simulink model "Final_V620140905h5b_fuben1"  (Simulink 7.9)
settings: Solver=FixedStepDiscrete  StartTime=0.0  StopTime=1  FixedStep=Auto  RelTol=1e-3
undefined symbols (not defined in the file or in its folder): Down, Up
libraries: tiiqmathlib x157, idelinklib_common x83, c2833xlib x37, simulink x12, c28xdmclib x12, c280xlib x7, simulink_extras x4, commutil2 x2, idelinklib_tgtpref x1, idelinklib_ticcs x1
(part 4 of 7)

== system Final_V620140905h5b_fuben1/action for state1 ==
  note: The fourth one is for load switch 0 is on
  note: The last one is for protect 0 is protect
  note: The sixth one is for Q2 on singal, 0 is on when the Q2 wants to be turned off, the i/o must be set to 1
  note: The third one is for Q2 off singal, 0 is off when the Q2 wants to be turned on, the i/o must be set to 1
  Action Port : ActionPort  ActionType=case
  Constant1 : Constant  Priority=1  Value=0  OutDataTypeStr=boolean
  Constant6 : Constant  Priority=1  Value=[1 1 1 1 1 0 1 1]  OutDataTypeStr=int8
  Digital Output : c2833xlib/Digital Output  Tag=1  Priority=2  GPIO_Number=GPIO8~GPIO15  GPIO_Bit0=off  GPIO_BIT0_Toggle=off  GPIO_Bit1=off  GPIO_BIT1_Toggle=off  GPIO_Bit2=off  GPIO_BIT2_Toggle=off  GPIO_Bit3=off  GPIO_BIT3_Toggle=off  GPIO_Bit4=on  GPIO_BIT4_Toggle=off  GPIO_Bit5=off  GPIO_BIT5_Toggle=off  GPIO_Bit6=off  GPIO_BIT6_Toggle=off  GPIO_Bit7=off  GPIO_BIT7_Toggle=off
  Out : Outport
  wires:
  Constant1/1 -> Digital Output/1
  Constant6/1 -> Out/1

== system Final_V620140905h5b_fuben1/action for state10 ==
  note: The third one is for Q2 off singal, 0 is off when the Q2 wants to be turned on, the i/o must be set to 1
  note: The sixth one is for Q2 on singal, 0 is on when the Q2 wants to be turned off, the i/o must be set to 1
  note: The last one is for protect 0 is protect
  note: The fourth one is for load switch 0 is on
  K : Inport
  Action Port : ActionPort  ActionType=case
  Constant1 : Constant  Priority=1  Value=0  OutDataTypeStr=boolean
  Constant3 : Constant  Priority=1  Value=[1 0 0 1 1 1 1 0]  OutDataTypeStr=int8
  Constant6 : Constant  Priority=1  Value=[1 1 1 1 1 1 1 0]  OutDataTypeStr=int8
  Digital Output : c2833xlib/Digital Output  Tag=1  Priority=2  GPIO_Number=GPIO8~GPIO15  GPIO_Bit0=off  GPIO_BIT0_Toggle=off  GPIO_Bit1=off  GPIO_BIT1_Toggle=off  GPIO_Bit2=off  GPIO_BIT2_Toggle=off  GPIO_Bit3=off  GPIO_BIT3_Toggle=off  GPIO_Bit4=on  GPIO_BIT4_Toggle=off  GPIO_Bit5=off  GPIO_BIT5_Toggle=off  GPIO_Bit6=off  GPIO_BIT6_Toggle=off  GPIO_Bit7=off  GPIO_BIT7_Toggle=off
  Switch1 : Switch  Criteria=u2 > Threshold  SaturateOnIntegerOverflow=on  InputSameDT=on
  Out : Outport
  wires:
  Constant1/1 -> Digital Output/1
  Switch1/1 -> Out/1
  K/1 -> Switch1/2
  Constant3/1 -> Switch1/1
  Constant6/1 -> Switch1/3

== system Final_V620140905h5b_fuben1/action for state11 ==
  note: The fourth one is for load switch 0 is on
  note: The last one is for protect 0 is protect
  note: The sixth one is for Q2 on singal, 0 is on when the Q2 wants to be turned off, the i/o must be set to 1
  note: The third one is for Q2 off singal, 0 is off when the Q2 wants to be turned on, the i/o must be set to 1
  Action Port : ActionPort  ActionType=case
  Constant1 : Constant  Priority=1  Value=0  OutDataTypeStr=boolean
  Constant6 : Constant  Priority=1  Value=[1 1 1 1 1 1 0 1]  OutDataTypeStr=int8
  Digital Output : c2833xlib/Digital Output  Tag=1  Priority=2  GPIO_Number=GPIO8~GPIO15  GPIO_Bit0=off  GPIO_BIT0_Toggle=off  GPIO_Bit1=off  GPIO_BIT1_Toggle=off  GPIO_Bit2=off  GPIO_BIT2_Toggle=off  GPIO_Bit3=off  GPIO_BIT3_Toggle=off  GPIO_Bit4=on  GPIO_BIT4_Toggle=off  GPIO_Bit5=off  GPIO_BIT5_Toggle=off  GPIO_Bit6=off  GPIO_BIT6_Toggle=off  GPIO_Bit7=off  GPIO_BIT7_Toggle=off
  Out : Outport
  wires:
  Constant1/1 -> Digital Output/1
  Constant6/1 -> Out/1

== system Final_V620140905h5b_fuben1/action for state12 ==
  note: The third one is for Q2 off singal, 0 is off when the Q2 wants to be turned on, the i/o must be set to 1
  note: The sixth one is for Q2 on singal, 0 is on when the Q2 wants to be turned off, the i/o must be set to 1
  note: The last one is for protect 0 is protect
  note: The fourth one is for load switch 0 is on
  Action Port : ActionPort  ActionType=case
  Constant1 : Constant  Priority=1  Value=0  OutDataTypeStr=boolean
  Constant6 : Constant  Priority=1  Value=[1 1 1 1 1 0 1 1]  OutDataTypeStr=int8
  Digital Output : c2833xlib/Digital Output  Tag=1  Priority=2  GPIO_Number=GPIO8~GPIO15  GPIO_Bit0=off  GPIO_BIT0_Toggle=off  GPIO_Bit1=off  GPIO_BIT1_Toggle=off  GPIO_Bit2=off  GPIO_BIT2_Toggle=off  GPIO_Bit3=off  GPIO_BIT3_Toggle=off  GPIO_Bit4=on  GPIO_BIT4_Toggle=off  GPIO_Bit5=off  GPIO_BIT5_Toggle=off  GPIO_Bit6=off  GPIO_BIT6_Toggle=off  GPIO_Bit7=off  GPIO_BIT7_Toggle=off
  Out : Outport
  wires:
  Constant1/1 -> Digital Output/1
  Constant6/1 -> Out/1

== system Final_V620140905h5b_fuben1/action for state2 ==
  note: The fourth one is for load switch 0 is on
  note: The last one is for protect 0 is protect
  note: The sixth one is for Q2 on singal, 0 is on when the Q2 wants to be turned off, the i/o must be set to 1
  note: The third one is for Q2 off singal, 0 is off when the Q2 wants to be turned on, the i/o must be set to 1
  Action Port : ActionPort  ActionType=case
  Constant1 : Constant  Priority=1  Value=0  OutDataTypeStr=boolean
  Constant6 : Constant  Priority=1  Value=[1 1 1 1 1 0 1 1]  OutDataTypeStr=int8
  Digital Output : c2833xlib/Digital Output  Tag=1  Priority=2  GPIO_Number=GPIO8~GPIO15  GPIO_Bit0=off  GPIO_BIT0_Toggle=off  GPIO_Bit1=off  GPIO_BIT1_Toggle=off  GPIO_Bit2=off  GPIO_BIT2_Toggle=off  GPIO_Bit3=off  GPIO_BIT3_Toggle=off  GPIO_Bit4=on  GPIO_BIT4_Toggle=off  GPIO_Bit5=off  GPIO_BIT5_Toggle=off  GPIO_Bit6=off  GPIO_BIT6_Toggle=off  GPIO_Bit7=off  GPIO_BIT7_Toggle=off
  Out : Outport
  wires:
  Constant1/1 -> Digital Output/1
  Constant6/1 -> Out/1

== system Final_V620140905h5b_fuben1/action for state3 ==
  note: The fourth one is for load switch 0 is on
  note: The last one is for protect 0 is protect
  note: The sixth one is for Q2 on singal, 0 is on when the Q2 wants to be turned off, the i/o must be set to 1
  note: The third one is for Q2 off singal, 0 is off when the Q2 wants to be turned on, the i/o must be set to 1
  Action Port : ActionPort  ActionType=case
  Constant1 : Constant  Priority=1  Value=0  OutDataTypeStr=boolean
  Constant6 : Constant  Priority=1  Value=[1 1 1 1 1 0 0 1]  OutDataTypeStr=int8
  Digital Output : c2833xlib/Digital Output  Tag=1  Priority=2  GPIO_Number=GPIO8~GPIO15  GPIO_Bit0=off  GPIO_BIT0_Toggle=off  GPIO_Bit1=off  GPIO_BIT1_Toggle=off  GPIO_Bit2=off  GPIO_BIT2_Toggle=off  GPIO_Bit3=off  GPIO_BIT3_Toggle=off  GPIO_Bit4=on  GPIO_BIT4_Toggle=off  GPIO_Bit5=off  GPIO_BIT5_Toggle=off  GPIO_Bit6=off  GPIO_BIT6_Toggle=off  GPIO_Bit7=off  GPIO_BIT7_Toggle=off
  Out : Outport
  wires:
  Constant1/1 -> Digital Output/1
  Constant6/1 -> Out/1

== system Final_V620140905h5b_fuben1/action for state5 ==
  note: Bit0:Fault=0
      | Bit1:G Connect to bus = 0
      | Bit2:
      | Bit3.Bit4:Lock switch = 0
      | Bit
  K : Inport
  Action Port : ActionPort  ActionType=case
  Constant1 : Constant  Priority=1  Value=0  OutDataTypeStr=boolean
  Constant3 : Constant  Priority=1  Value=[1 0 0 0 0 0 0 1]  OutDataTypeStr=int8
  Constant6 : Constant  Priority=1  Value=[1 1 1 0 0 0 0 1]  OutDataTypeStr=int8
  Digital Output : c2833xlib/Digital Output  Tag=1  Priority=2  GPIO_Number=GPIO8~GPIO15  GPIO_Bit0=off  GPIO_BIT0_Toggle=off  GPIO_Bit1=off  GPIO_BIT1_Toggle=off  GPIO_Bit2=off  GPIO_BIT2_Toggle=off  GPIO_Bit3=off  GPIO_BIT3_Toggle=off  GPIO_Bit4=on  GPIO_BIT4_Toggle=off  GPIO_Bit5=off  GPIO_BIT5_Toggle=off  GPIO_Bit6=off  GPIO_BIT6_Toggle=off  GPIO_Bit7=off  GPIO_BIT7_Toggle=off
  Switch1 : Switch  Criteria=u2 > Threshold  SaturateOnIntegerOverflow=on  InputSameDT=on
  Out : Outport
  wires:
  Constant1/1 -> Digital Output/1
  Switch1/1 -> Out/1
  K/1 -> Switch1/2
  Constant3/1 -> Switch1/1
  Constant6/1 -> Switch1/3

== system Final_V620140905h5b_fuben1/action for state6 ==
  note: The fourth one is for load switch 0 is on
  note: The last one is for protect 0 is protect
  note: The sixth one is for Q2 on singal, 0 is on when the Q2 wants to be turned off, the i/o must be set to 1
  note: The third one is for Q2 off singal, 0 is off when the Q2 wants to be turned on, the i/o must be set to 1
  Action Port : ActionPort  ActionType=case
  Constant1 : Constant  Priority=1  Value=0  OutDataTypeStr=boolean
  Constant6 : Constant  Priority=1  Value=[1 1 1 0 0 1 0 1]  OutDataTypeStr=int8
  Digital Output : c2833xlib/Digital Output  Tag=1  Priority=2  GPIO_Number=GPIO8~GPIO15  GPIO_Bit0=off  GPIO_BIT0_Toggle=off  GPIO_Bit1=off  GPIO_BIT1_Toggle=off  GPIO_Bit2=off  GPIO_BIT2_Toggle=off  GPIO_Bit3=off  GPIO_BIT3_Toggle=off  GPIO_Bit4=on  GPIO_BIT4_Toggle=off  GPIO_Bit5=off  GPIO_BIT5_Toggle=off  GPIO_Bit6=off  GPIO_BIT6_Toggle=off  GPIO_Bit7=off  GPIO_BIT7_Toggle=off
  Out : Outport
  wires:
  Constant1/1 -> Digital Output/1
  Constant6/1 -> Out/1

== system Final_V620140905h5b_fuben1/action for state7 ==
  note: The fourth one is for load switch 0 is on
  note: The last one is for protect 0 is protect
  note: The sixth one is for Q2 on singal, 0 is on when the Q2 wants to be turned off, the i/o must be set to 1
  note: The third one is for Q2 off singal, 0 is off when the Q2 wants to be turned on, the i/o must be set to 1
  Action Port : ActionPort  ActionType=case
  Constant1 : Constant  Priority=1  Value=0  OutDataTypeStr=boolean
  Constant6 : Constant  Priority=1  Value=[1 1 1 0 0 1 0 1]  OutDataTypeStr=int8
  Digital Output : c2833xlib/Digital Output  Tag=1  Priority=2  GPIO_Number=GPIO8~GPIO15  GPIO_Bit0=off  GPIO_BIT0_Toggle=off  GPIO_Bit1=off  GPIO_BIT1_Toggle=off  GPIO_Bit2=off  GPIO_BIT2_Toggle=off  GPIO_Bit3=off  GPIO_BIT3_Toggle=off  GPIO_Bit4=on  GPIO_BIT4_Toggle=off  GPIO_Bit5=off  GPIO_BIT5_Toggle=off  GPIO_Bit6=off  GPIO_BIT6_Toggle=off  GPIO_Bit7=off  GPIO_BIT7_Toggle=off
  Out : Outport
  wires:
  Constant1/1 -> Digital Output/1
  Constant6/1 -> Out/1

== system Final_V620140905h5b_fuben1/action for state8 ==
  note: The third one is for Q2 off singal, 0 is off when the Q2 wants to be turned on, the i/o must be set to 1
  note: The sixth one is for Q2 on singal, 0 is on when the Q2 wants to be turned off, the i/o must be set to 1
  note: The last one is for protect 0 is protect
  note: The fourth one is for load switch 0 is on
  Action Port : ActionPort  ActionType=case
  Constant1 : Constant  Priority=1  Value=0  OutDataTypeStr=boolean
  Constant5 : Constant  Priority=1  Value=[1 1 1 1 1 0 0 1]  OutDataTypeStr=int8
  Digital Output : c2833xlib/Digital Output  Tag=1  Priority=2  GPIO_Number=GPIO8~GPIO15  GPIO_Bit0=off  GPIO_BIT0_Toggle=off  GPIO_Bit1=off  GPIO_BIT1_Toggle=off  GPIO_Bit2=off  GPIO_BIT2_Toggle=off  GPIO_Bit3=off  GPIO_BIT3_Toggle=off  GPIO_Bit4=on  GPIO_BIT4_Toggle=off  GPIO_Bit5=off  GPIO_BIT5_Toggle=off  GPIO_Bit6=off  GPIO_BIT6_Toggle=off  GPIO_Bit7=off  GPIO_BIT7_Toggle=off
  Out : Outport
  wires:
  Constant1/1 -> Digital Output/1
  Constant5/1 -> Out/1

== system Final_V620140905h5b_fuben1/action for state9 ==
  note: The fourth one is for load switch 0 is on
  note: The last one is for protect 0 is protect
  note: The sixth one is for Q2 on singal, 0 is on when the Q2 wants to be turned off, the i/o must be set to 1
  note: The third one is for Q2 off singal, 0 is off when the Q2 wants to be turned on, the i/o must be set to 1
  Action Port : ActionPort  ActionType=case
  Constant1 : Constant  Priority=1  Value=0  OutDataTypeStr=boolean
  Constant6 : Constant  Priority=1  Value=[1 1 1 1 1 0 1 1]  OutDataTypeStr=int8
  Digital Output : c2833xlib/Digital Output  Tag=1  Priority=2  GPIO_Number=GPIO8~GPIO15  GPIO_Bit0=off  GPIO_BIT0_Toggle=off  GPIO_Bit1=off  GPIO_BIT1_Toggle=off  GPIO_Bit2=off  GPIO_BIT2_Toggle=off  GPIO_Bit3=off  GPIO_BIT3_Toggle=off  GPIO_Bit4=on  GPIO_BIT4_Toggle=off  GPIO_Bit5=off  GPIO_BIT5_Toggle=off  GPIO_Bit6=off  GPIO_BIT6_Toggle=off  GPIO_Bit7=off  GPIO_BIT7_Toggle=off
  Out : Outport
  wires:
  Constant1/1 -> Digital Output/1
  Constant6/1 -> Out/1

== system Final_V620140905h5b_fuben1/actrion for state4 ==
  note: The fourth one is for load switch 0 is on
  note: The last one is for protect 0 is protect
  note: The sixth one is for Q2 on singal, 0 is on when the Q2 wants to be turned off, the i/o must be set to 1
  note: The third one is for Q2 off singal, 0 is off when the Q2 wants to be turned on, the i/o must be set to 1
  K : Inport
  Action Port : ActionPort  ActionType=case
  Constant1 : Constant  Priority=1  Value=0  OutDataTypeStr=boolean
  Constant2 : Constant  Priority=1  Value=[1 0 0 0 0 1 0 1]  OutDataTypeStr=int8
  Constant6 : Constant  Priority=1  Value=[1 1 1 0 0 1 0 1]  OutDataTypeStr=int8
  Digital Output : c2833xlib/Digital Output  Tag=1  Priority=2  GPIO_Number=GPIO8~GPIO15  GPIO_Bit0=off  GPIO_BIT0_Toggle=off  GPIO_Bit1=off  GPIO_BIT1_Toggle=off  GPIO_Bit2=off  GPIO_BIT2_Toggle=off  GPIO_Bit3=off  GPIO_BIT3_Toggle=off  GPIO_Bit4=on  GPIO_BIT4_Toggle=off  GPIO_Bit5=off  GPIO_BIT5_Toggle=off  GPIO_Bit6=off  GPIO_BIT6_Toggle=off  GPIO_Bit7=off  GPIO_BIT7_Toggle=off
  Switch1 : Switch  Criteria=u2 > Threshold  SaturateOnIntegerOverflow=on  InputSameDT=on
  Out : Outport
  wires:
  Constant1/1 -> Digital Output/1
  K/1 -> Switch1/2
  Constant6/1 -> Switch1/3
  Switch1/1 -> Out/1
  Constant2/1 -> Switch1/1

== system Final_V620140905h5b_fuben1/Function-Call Subsystem1/0 ==
  Action Port : ActionPort  ActionType=case
  Constant{1,3..4,7..8} (5 alike) : Constant  Priority=1  Value=0  OutDataTypeStr=boolean
  Constant2 : Constant  Priority=1  OutDataTypeStr=boolean
  Constant5 : Constant  Priority=1  OutDataTypeStr=boolean
  Constant6 : Constant  Priority=1  OutDataTypeStr=boolean
  Mux : Mux  Inputs=8
  Out1 : Outport
  wires:
  Constant2/1 -> Mux/1
  Constant1/1 -> Mux/2
  Constant3/1 -> Mux/3
  Constant4/1 -> Mux/4
  Constant5/1 -> Mux/5
  Constant6/1 -> Mux/6
  Constant7/1 -> Mux/7
  Constant8/1 -> Mux/8
  Mux/1 -> Out1/1

== system Final_V620140905h5b_fuben1/Function-Call Subsystem1/1 ==
  Action Port : ActionPort  ActionType=case
  Constant1 : Constant  Priority=1  OutDataTypeStr=boolean
  Constant{2..3,5..8} (6 alike) : Constant  Priority=1  Value=0  OutDataTypeStr=boolean
  Constant4 : Constant  Priority=1  OutDataTypeStr=boolean
  Mux : Mux  Inputs=8
  Out1 : Outport
  wires:
  Mux/1 -> Out1/1
  Constant8/1 -> Mux/8
  Constant7/1 -> Mux/7
  Constant6/1 -> Mux/6
  Constant5/1 -> Mux/5
  Constant4/1 -> Mux/4
  Constant3/1 -> Mux/3
  Constant1/1 -> Mux/2
  Constant2/1 -> Mux/1

== system Final_V620140905h5b_fuben1/Function-Call Subsystem1/10 ==
  Action Port : ActionPort  ActionType=case
  Constant{1,3..8} (7 alike) : Constant  Priority=1  Value=0  OutDataTypeStr=boolean
  Constant2 : Constant  Priority=1  OutDataTypeStr=boolean
  Mux : Mux  Inputs=8
  Out1 : Outport
  wires:
  Mux/1 -> Out1/1
  Constant8/1 -> Mux/8
  Constant7/1 -> Mux/7
  Constant6/1 -> Mux/6
  Constant5/1 -> Mux/5
  Constant4/1 -> Mux/4
  Constant3/1 -> Mux/3
  Constant1/1 -> Mux/2
  Constant2/1 -> Mux/1

== system Final_V620140905h5b_fuben1/Function-Call Subsystem1/11 ==
  Action Port : ActionPort  ActionType=case
  Constant{1,3..4,7} (4 alike) : Constant  Priority=1  OutDataTypeStr=boolean
  Constant{2,5..6,8} (4 alike) : Constant  Priority=1  Value=0  OutDataTypeStr=boolean
  Mux : Mux  Inputs=8
  Out1 : Outport
  wires:
  Constant2/1 -> Mux/1
  Constant1/1 -> Mux/2
  Constant3/1 -> Mux/3
  Constant4/1 -> Mux/4
  Constant5/1 -> Mux/5
  Constant6/1 -> Mux/6
  Constant7/1 -> Mux/7
  Constant8/1 -> Mux/8
  Mux/1 -> Out1/1

== system Final_V620140905h5b_fuben1/Function-Call Subsystem1/12 ==
  Action Port : ActionPort  ActionType=case
  Constant{1..2,5..8} (6 alike) : Constant  Priority=1  Value=0  OutDataTypeStr=boolean
  Constant3 : Constant  Priority=1  OutDataTypeStr=boolean
  Constant4 : Constant  Priority=1  OutDataTypeStr=boolean
  Mux : Mux  Inputs=8
  Out1 : Outport
  wires:
  Mux/1 -> Out1/1
  Constant8/1 -> Mux/8
  Constant7/1 -> Mux/7
  Constant6/1 -> Mux/6
  Constant5/1 -> Mux/5
  Constant4/1 -> Mux/4
  Constant3/1 -> Mux/3
  Constant1/1 -> Mux/2
  Constant2/1 -> Mux/1

== system Final_V620140905h5b_fuben1/Function-Call Subsystem1/2 ==
  Action Port : ActionPort  ActionType=case
  Constant{1,3..4,7} (4 alike) : Constant  Priority=1  OutDataTypeStr=boolean
  Constant{2,5..6,8} (4 alike) : Constant  Priority=1  Value=0  OutDataTypeStr=boolean
  Mux : Mux  Inputs=8
  Out1 : Outport
  wires:
  Constant2/1 -> Mux/1
  Constant1/1 -> Mux/2
  Constant3/1 -> Mux/3
  Constant4/1 -> Mux/4
  Constant5/1 -> Mux/5
  Constant6/1 -> Mux/6
  Constant7/1 -> Mux/7
  Constant8/1 -> Mux/8
  Mux/1 -> Out1/1

== system Final_V620140905h5b_fuben1/Function-Call Subsystem1/3 ==
  Action Port : ActionPort  ActionType=case
  Constant{1,3..4,7} (4 alike) : Constant  Priority=1  OutDataTypeStr=boolean
  Constant{2,5..6,8} (4 alike) : Constant  Priority=1  Value=0  OutDataTypeStr=boolean
  Mux : Mux  Inputs=8
  Out1 : Outport
  wires:
  Mux/1 -> Out1/1
  Constant8/1 -> Mux/8
  Constant7/1 -> Mux/7
  Constant6/1 -> Mux/6
  Constant5/1 -> Mux/5
  Constant4/1 -> Mux/4
  Constant3/1 -> Mux/3
  Constant1/1 -> Mux/2
  Constant2/1 -> Mux/1

== system Final_V620140905h5b_fuben1/Function-Call Subsystem1/4 ==
  Action Port : ActionPort  ActionType=case
  Constant{1..3,5..8} (7 alike) : Constant  Priority=1  Value=0  OutDataTypeStr=boolean
  Constant4 : Constant  Priority=1  OutDataTypeStr=boolean
  Mux : Mux  Inputs=8
  Out1 : Outport
  wires:
  Constant2/1 -> Mux/1
  Constant1/1 -> Mux/2
  Constant3/1 -> Mux/3
  Constant4/1 -> Mux/4
  Constant5/1 -> Mux/5
  Constant6/1 -> Mux/6
  Constant7/1 -> Mux/7
  Constant8/1 -> Mux/8
  Mux/1 -> Out1/1

== system Final_V620140905h5b_fuben1/Function-Call Subsystem1/5 ==
  Action Port : ActionPort  ActionType=case
  Constant{1..3,5..6,8} (6 alike) : Constant  Priority=1  Value=0  OutDataTypeStr=boolean
  Constant4 : Constant  Priority=1  OutDataTypeStr=boolean
  Constant7 : Constant  Priority=1  OutDataTypeStr=boolean
  Mux : Mux  Inputs=8
  Out1 : Outport
  wires:
  Mux/1 -> Out1/1
  Constant8/1 -> Mux/8
  Constant7/1 -> Mux/7
  Constant6/1 -> Mux/6
  Constant5/1 -> Mux/5
  Constant4/1 -> Mux/4
  Constant3/1 -> Mux/3
  Constant1/1 -> Mux/2
  Constant2/1 -> Mux/1

== system Final_V620140905h5b_fuben1/Function-Call Subsystem1/6 ==
  Action Port : ActionPort  ActionType=case
  Constant1 : Constant  Priority=1  OutDataTypeStr=boolean
  Constant{2,5..8} (5 alike) : Constant  Priority=1  Value=0  OutDataTypeStr=boolean
  Constant3 : Constant  Priority=1  OutDataTypeStr=boolean
  Constant4 : Constant  Priority=1  OutDataTypeStr=boolean
  Mux : Mux  Inputs=8
  Out1 : Outport
  wires:
  Mux/1 -> Out1/1
  Constant8/1 -> Mux/8
  Constant7/1 -> Mux/7
  Constant6/1 -> Mux/6
  Constant5/1 -> Mux/5
  Constant4/1 -> Mux/4
  Constant3/1 -> Mux/3
  Constant1/1 -> Mux/2
  Constant2/1 -> Mux/1

== system Final_V620140905h5b_fuben1/Function-Call Subsystem1/7 ==
  Action Port : ActionPort  ActionType=case
  Constant{1,3..4,7} (4 alike) : Constant  Priority=1  OutDataTypeStr=boolean
  Constant{2,5..6,8} (4 alike) : Constant  Priority=1  Value=0  OutDataTypeStr=boolean
  Mux : Mux  Inputs=8
  Out1 : Outport
  wires:
  Constant2/1 -> Mux/1
  Constant1/1 -> Mux/2
  Constant3/1 -> Mux/3
  Constant4/1 -> Mux/4
  Constant5/1 -> Mux/5
  Constant6/1 -> Mux/6
  Constant7/1 -> Mux/7
  Constant8/1 -> Mux/8
  Mux/1 -> Out1/1

== system Final_V620140905h5b_fuben1/Function-Call Subsystem1/8 ==
  Action Port : ActionPort  ActionType=case
  Constant{1,3..4,7} (4 alike) : Constant  Priority=1  OutDataTypeStr=boolean
  Constant{2,5..6,8} (4 alike) : Constant  Priority=1  Value=0  OutDataTypeStr=boolean
  Mux : Mux  Inputs=8
  Out1 : Outport
  wires:
  Mux/1 -> Out1/1
  Constant8/1 -> Mux/8
  Constant7/1 -> Mux/7
  Constant6/1 -> Mux/6
  Constant5/1 -> Mux/5
  Constant4/1 -> Mux/4
  Constant3/1 -> Mux/3
  Constant1/1 -> Mux/2
  Constant2/1 -> Mux/1

== system Final_V620140905h5b_fuben1/Function-Call Subsystem1/9 ==
  Action Port : ActionPort  ActionType=case
  Constant{1..3,5..6,8} (6 alike) : Constant  Priority=1  Value=0  OutDataTypeStr=boolean
  Constant4 : Constant  Priority=1  OutDataTypeStr=boolean
  Constant7 : Constant  Priority=1  OutDataTypeStr=boolean
  Mux : Mux  Inputs=8
  Out1 : Outport
  wires:
  Constant2/1 -> Mux/1
  Constant1/1 -> Mux/2
  Constant3/1 -> Mux/3
  Constant4/1 -> Mux/4
  Constant5/1 -> Mux/5
  Constant6/1 -> Mux/6
  Constant7/1 -> Mux/7
  Constant8/1 -> Mux/8
  Mux/1 -> Out1/1

== system Final_V620140905h5b_fuben1/Function-Call Subsystem1/AD ==
  Read AD : Subsystem  Priority=2
  Start Conversion : Subsystem  Priority=1
  Stop Conversion : Subsystem  Priority=3

== system Final_V620140905h5b_fuben1/Function-Call Subsystem1/Current protect ==
  igdin : Inport
  Reset : Inport  Port=2
  Constant25 : Constant  Value=0  OutDataTypeStr=boolean
  Constant26 : Constant  OutDataTypeStr=boolean
  S-R Flip-Flop1 : simulink_extras/Flip Flops/S-R Flip-Flop  initial_condition=0
  Switch9 : Switch  Criteria=u2 > Threshold  Threshold=380  SaturateOnIntegerOverflow=on  InputSameDT=on
  Terminator : Terminator
  Software_I : Outport
  wires:
  Constant26/1 -> Switch9/1
  Constant25/1 -> Switch9/3
  S-R Flip-Flop1/1 -> Software_I/1
  Reset/1 -> S-R Flip-Flop1/2
  S-R Flip-Flop1/2 -> Terminator/1
  Switch9/1 -> S-R Flip-Flop1/1
  igdin/1 -> Switch9/2

== system Final_V620140905h5b_fuben1/Function-Call Subsystem1/Current protect1 ==
  igdin : Inport
  Reset : Inport  Port=2
  Constant25 : Constant  Value=0  OutDataTypeStr=boolean
  Constant26 : Constant  OutDataTypeStr=boolean
  S-R Flip-Flop1 : simulink_extras/Flip Flops/S-R Flip-Flop  initial_condition=0
  Switch9 : Switch  Criteria=u2 > Threshold  Threshold=350  SaturateOnIntegerOverflow=on  InputSameDT=on
  Terminator : Terminator
  Software_I : Outport
  wires:
  igdin/1 -> Switch9/2
  Switch9/1 -> S-R Flip-Flop1/1
  S-R Flip-Flop1/2 -> Terminator/1
  Reset/1 -> S-R Flip-Flop1/2
  S-R Flip-Flop1/1 -> Software_I/1
  Constant25/1 -> Switch9/3
  Constant26/1 -> Switch9/1

== system Final_V620140905h5b_fuben1/Function-Call Subsystem1/ION multiply1 ==
  x : Inport
  Constant2 : Constant  Value=x  OutDataTypeStr=fixdt(1,32,16)
  IQN x IQN : tiiqmathlib/IQN x IQN  multiplyOption=Multiply
  Kx : Outport
  wires:
  IQN x IQN/1 -> Kx/1
  x/1 -> IQN x IQN/1
  Constant2/1 -> IQN x IQN/2

== system Final_V620140905h5b_fuben1/Function-Call Subsystem1/ION multiply10 ==
  x : Inport
  Constant2 : Constant  Value=x  OutDataTypeStr=fixdt(1,32,16)
  IQN x IQN : tiiqmathlib/IQN x IQN  multiplyOption=Multiply
  Kx : Outport
  wires:
  IQN x IQN/1 -> Kx/1
  x/1 -> IQN x IQN/1
  Constant2/1 -> IQN x IQN/2

== system Final_V620140905h5b_fuben1/Function-Call Subsystem1/ION multiply11 ==
  x : Inport
  Constant2 : Constant  Value=x  OutDataTypeStr=fixdt(1,32,16)
  IQN x IQN : tiiqmathlib/IQN x IQN  multiplyOption=Multiply
  Kx : Outport
  wires:
  Constant2/1 -> IQN x IQN/2
  x/1 -> IQN x IQN/1
  IQN x IQN/1 -> Kx/1

== system Final_V620140905h5b_fuben1/Function-Call Subsystem1/ION multiply12 ==
  x : Inport
  Constant2 : Constant  Value=x  OutDataTypeStr=fixdt(1,32,16)
  IQN x IQN : tiiqmathlib/IQN x IQN  multiplyOption=Multiply
  Kx : Outport
  wires:
  Constant2/1 -> IQN x IQN/2
  x/1 -> IQN x IQN/1
  IQN x IQN/1 -> Kx/1

== system Final_V620140905h5b_fuben1/Function-Call Subsystem1/ION multiply13 ==
  x : Inport
  Constant2 : Constant  Value=x  OutDataTypeStr=fixdt(1,32,16)
  IQN x IQN : tiiqmathlib/IQN x IQN  multiplyOption=Multiply
  Kx : Outport
  wires:
  Constant2/1 -> IQN x IQN/2
  x/1 -> IQN x IQN/1
  IQN x IQN/1 -> Kx/1

== system Final_V620140905h5b_fuben1/Function-Call Subsystem1/ION multiply14 ==
  x : Inport
  Constant2 : Constant  Value=x  OutDataTypeStr=fixdt(1,32,16)
  IQN x IQN : tiiqmathlib/IQN x IQN  multiplyOption=Multiply
  Kx : Outport
  wires:
  IQN x IQN/1 -> Kx/1
  x/1 -> IQN x IQN/1
  Constant2/1 -> IQN x IQN/2

== system Final_V620140905h5b_fuben1/Function-Call Subsystem1/ION multiply15 ==
  x : Inport
  Constant2 : Constant  Value=x  OutDataTypeStr=fixdt(1,32,16)
  IQN x IQN : tiiqmathlib/IQN x IQN  multiplyOption=Multiply
  Kx : Outport
  wires:
  IQN x IQN/1 -> Kx/1
  x/1 -> IQN x IQN/1
  Constant2/1 -> IQN x IQN/2

== system Final_V620140905h5b_fuben1/Function-Call Subsystem1/ION multiply16 ==
  x : Inport
  Constant2 : Constant  Value=x  OutDataTypeStr=fixdt(1,32,16)
  IQN x IQN : tiiqmathlib/IQN x IQN  multiplyOption=Multiply
  Kx : Outport
  wires:
  IQN x IQN/1 -> Kx/1
  x/1 -> IQN x IQN/1
  Constant2/1 -> IQN x IQN/2

== system Final_V620140905h5b_fuben1/Function-Call Subsystem1/ION multiply17 ==
  x : Inport
  Constant2 : Constant  Value=x  OutDataTypeStr=fixdt(1,32,16)
  IQN x IQN : tiiqmathlib/IQN x IQN  multiplyOption=Multiply
  Kx : Outport
  wires:
  IQN x IQN/1 -> Kx/1
  x/1 -> IQN x IQN/1
  Constant2/1 -> IQN x IQN/2

== system Final_V620140905h5b_fuben1/Function-Call Subsystem1/ION multiply19 ==
  x : Inport
  Constant2 : Constant  Value=x  OutDataTypeStr=fixdt(1,32,16)
  IQN x IQN : tiiqmathlib/IQN x IQN  multiplyOption=Multiply
  Kx : Outport
  wires:
  IQN x IQN/1 -> Kx/1
  x/1 -> IQN x IQN/1
  Constant2/1 -> IQN x IQN/2

== system Final_V620140905h5b_fuben1/Function-Call Subsystem1/ION multiply2 ==
  x : Inport
  Constant2 : Constant  Value=x  OutDataTypeStr=fixdt(1,32,16)
  IQN x IQN : tiiqmathlib/IQN x IQN  multiplyOption=Multiply
  Kx : Outport
  wires:
  IQN x IQN/1 -> Kx/1
  x/1 -> IQN x IQN/1
  Constant2/1 -> IQN x IQN/2

== system Final_V620140905h5b_fuben1/Function-Call Subsystem1/ION multiply20 ==
  x : Inport
  Constant2 : Constant  Value=x  OutDataTypeStr=fixdt(1,32,16)
  IQN x IQN : tiiqmathlib/IQN x IQN  multiplyOption=Multiply
  Kx : Outport
  wires:
  Constant2/1 -> IQN x IQN/2
  x/1 -> IQN x IQN/1
  IQN x IQN/1 -> Kx/1

== system Final_V620140905h5b_fuben1/Function-Call Subsystem1/ION multiply21 ==
  x : Inport
  Constant2 : Constant  Value=x  OutDataTypeStr=fixdt(1,32,16)
  IQN x IQN : tiiqmathlib/IQN x IQN  multiplyOption=Multiply
  Kx : Outport
  wires:
  IQN x IQN/1 -> Kx/1
  x/1 -> IQN x IQN/1
  Constant2/1 -> IQN x IQN/2

== system Final_V620140905h5b_fuben1/Function-Call Subsystem1/ION multiply22 ==
  x : Inport
  Constant2 : Constant  Value=x  OutDataTypeStr=fixdt(1,32,16)
  IQN x IQN : tiiqmathlib/IQN x IQN  multiplyOption=Multiply
  Kx : Outport
  wires:
  IQN x IQN/1 -> Kx/1
  x/1 -> IQN x IQN/1
  Constant2/1 -> IQN x IQN/2

== system Final_V620140905h5b_fuben1/Function-Call Subsystem1/ION multiply23 ==
  x : Inport
  Constant2 : Constant  Value=x  OutDataTypeStr=fixdt(1,32,16)
  IQN x IQN : tiiqmathlib/IQN x IQN  multiplyOption=Multiply
  Kx : Outport
  wires:
  Constant2/1 -> IQN x IQN/2
  x/1 -> IQN x IQN/1
  IQN x IQN/1 -> Kx/1

== system Final_V620140905h5b_fuben1/Function-Call Subsystem1/ION multiply24 ==
  x : Inport
  Constant2 : Constant  Value=x  OutDataTypeStr=fixdt(1,32,16)
  IQN x IQN : tiiqmathlib/IQN x IQN  multiplyOption=Multiply
  Kx : Outport
  wires:
  IQN x IQN/1 -> Kx/1
  x/1 -> IQN x IQN/1
  Constant2/1 -> IQN x IQN/2

== system Final_V620140905h5b_fuben1/Function-Call Subsystem1/ION multiply25 ==
  x : Inport
  Constant2 : Constant  Value=x  OutDataTypeStr=fixdt(1,32,16)
  IQN x IQN : tiiqmathlib/IQN x IQN  multiplyOption=Multiply
  Kx : Outport
  wires:
  Constant2/1 -> IQN x IQN/2
  x/1 -> IQN x IQN/1
  IQN x IQN/1 -> Kx/1

== system Final_V620140905h5b_fuben1/Function-Call Subsystem1/ION multiply26 ==
  x : Inport
  Constant2 : Constant  Value=x  OutDataTypeStr=fixdt(1,32,16)
  IQN x IQN : tiiqmathlib/IQN x IQN  multiplyOption=Multiply
  Kx : Outport
  wires:
  IQN x IQN/1 -> Kx/1
  x/1 -> IQN x IQN/1
  Constant2/1 -> IQN x IQN/2

== system Final_V620140905h5b_fuben1/Function-Call Subsystem1/ION multiply27 ==
  x : Inport
  Constant2 : Constant  Value=x  OutDataTypeStr=fixdt(1,32,16)
  IQN x IQN : tiiqmathlib/IQN x IQN  multiplyOption=Multiply
  Kx : Outport
  wires:
  IQN x IQN/1 -> Kx/1
  x/1 -> IQN x IQN/1
  Constant2/1 -> IQN x IQN/2

== system Final_V620140905h5b_fuben1/Function-Call Subsystem1/ION multiply28 ==
  x : Inport
  Constant2 : Constant  Value=x  OutDataTypeStr=fixdt(1,32,16)
  IQN x IQN : tiiqmathlib/IQN x IQN  multiplyOption=Multiply
  Kx : Outport
  wires:
  Constant2/1 -> IQN x IQN/2
  x/1 -> IQN x IQN/1
  IQN x IQN/1 -> Kx/1

== system Final_V620140905h5b_fuben1/Function-Call Subsystem1/ION multiply29 ==
  x : Inport
  Constant2 : Constant  Value=x  OutDataTypeStr=fixdt(1,32,16)
  IQN x IQN : tiiqmathlib/IQN x IQN  multiplyOption=Multiply
  Kx : Outport
  wires:
  Constant2/1 -> IQN x IQN/2
  x/1 -> IQN x IQN/1
  IQN x IQN/1 -> Kx/1

== system Final_V620140905h5b_fuben1/Function-Call Subsystem1/ION multiply3 ==
  x : Inport
  Constant2 : Constant  Value=x  OutDataTypeStr=fixdt(1,32,16)
  IQN x IQN : tiiqmathlib/IQN x IQN  multiplyOption=Multiply
  Kx : Outport
  wires:
  Constant2/1 -> IQN x IQN/2
  x/1 -> IQN x IQN/1
  IQN x IQN/1 -> Kx/1

== system Final_V620140905h5b_fuben1/Function-Call Subsystem1/ION multiply30 ==
  x : Inport
  Constant2 : Constant  Value=x  OutDataTypeStr=fixdt(1,32,16)
  IQN x IQN : tiiqmathlib/IQN x IQN  multiplyOption=Multiply
  Kx : Outport
  wires:
  IQN x IQN/1 -> Kx/1
  x/1 -> IQN x IQN/1
  Constant2/1 -> IQN x IQN/2

== system Final_V620140905h5b_fuben1/Function-Call Subsystem1/ION multiply31 ==
  x : Inport
  Constant2 : Constant  Value=x  OutDataTypeStr=fixdt(1,32,16)
  IQN x IQN : tiiqmathlib/IQN x IQN  multiplyOption=Multiply
  Kx : Outport
  wires:
  IQN x IQN/1 -> Kx/1
  x/1 -> IQN x IQN/1
  Constant2/1 -> IQN x IQN/2

== system Final_V620140905h5b_fuben1/Function-Call Subsystem1/ION multiply32 ==
  x : Inport
  Constant2 : Constant  Value=x  OutDataTypeStr=fixdt(1,32,16)
  IQN x IQN : tiiqmathlib/IQN x IQN  multiplyOption=Multiply
  Kx : Outport
  wires:
  Constant2/1 -> IQN x IQN/2
  x/1 -> IQN x IQN/1
  IQN x IQN/1 -> Kx/1

== system Final_V620140905h5b_fuben1/Function-Call Subsystem1/ION multiply33 ==
  x : Inport
  Constant2 : Constant  Value=x  OutDataTypeStr=fixdt(1,32,16)
  IQN x IQN : tiiqmathlib/IQN x IQN  multiplyOption=Multiply
  Kx : Outport
  wires:
  Constant2/1 -> IQN x IQN/2
  x/1 -> IQN x IQN/1
  IQN x IQN/1 -> Kx/1

== system Final_V620140905h5b_fuben1/Function-Call Subsystem1/ION multiply34 ==
  x : Inport
  Constant2 : Constant  Value=x  OutDataTypeStr=fixdt(1,32,16)
  IQN x IQN : tiiqmathlib/IQN x IQN  multiplyOption=Multiply
  Kx : Outport
  wires:
  Constant2/1 -> IQN x IQN/2
  x/1 -> IQN x IQN/1
  IQN x IQN/1 -> Kx/1

== system Final_V620140905h5b_fuben1/Function-Call Subsystem1/ION multiply35 ==
  x : Inport
  Constant2 : Constant  Value=x  OutDataTypeStr=fixdt(1,32,16)
  IQN x IQN : tiiqmathlib/IQN x IQN  multiplyOption=Multiply
  Kx : Outport
  wires:
  IQN x IQN/1 -> Kx/1
  x/1 -> IQN x IQN/1
  Constant2/1 -> IQN x IQN/2

== system Final_V620140905h5b_fuben1/Function-Call Subsystem1/ION multiply36 ==
  x : Inport
  Constant2 : Constant  Value=x  OutDataTypeStr=fixdt(1,32,16)
  IQN x IQN : tiiqmathlib/IQN x IQN  multiplyOption=Multiply
  Kx : Outport
  wires:
  IQN x IQN/1 -> Kx/1
  x/1 -> IQN x IQN/1
  Constant2/1 -> IQN x IQN/2

== system Final_V620140905h5b_fuben1/Function-Call Subsystem1/ION multiply39 ==
  x : Inport
  Constant2 : Constant  Value=x  OutDataTypeStr=Inherit: Inherit via back propagation
  IQN x IQN : tiiqmathlib/IQN x IQN  multiplyOption=Multiply
  Kx : Outport
  wires:
  IQN x IQN/1 -> Kx/1
  x/1 -> IQN x IQN/1
  Constant2/1 -> IQN x IQN/2

== system Final_V620140905h5b_fuben1/Function-Call Subsystem1/ION multiply4 ==
  x : Inport
  Constant2 : Constant  Value=x  OutDataTypeStr=fixdt(1,32,16)
  IQN x IQN : tiiqmathlib/IQN x IQN  multiplyOption=Multiply
  Kx : Outport
  wires:
  IQN x IQN/1 -> Kx/1
  x/1 -> IQN x IQN/1
  Constant2/1 -> IQN x IQN/2

== system Final_V620140905h5b_fuben1/Function-Call Subsystem1/ION multiply44 ==
  x : Inport
  Constant2 : Constant  Value=x  OutDataTypeStr=fixdt(1,32,16)
  IQN x IQN : tiiqmathlib/IQN x IQN  multiplyOption=Multiply
  Kx : Outport
  wires:
  IQN x IQN/1 -> Kx/1
  x/1 -> IQN x IQN/1
  Constant2/1 -> IQN x IQN/2

== system Final_V620140905h5b_fuben1/Function-Call Subsystem1/ION multiply45 ==
  x : Inport
  Constant2 : Constant  Value=x  OutDataTypeStr=fixdt(1,32,16)
  IQN x IQN : tiiqmathlib/IQN x IQN  multiplyOption=Multiply
  Kx : Outport
  wires:
  Constant2/1 -> IQN x IQN/2
  x/1 -> IQN x IQN/1
  IQN x IQN/1 -> Kx/1

== system Final_V620140905h5b_fuben1/Function-Call Subsystem1/ION multiply46 ==
  x : Inport
  Constant2 : Constant  Value=x  OutDataTypeStr=fixdt(1,32,16)
  IQN x IQN : tiiqmathlib/IQN x IQN  multiplyOption=Multiply
  Kx : Outport
  wires:
  Constant2/1 -> IQN x IQN/2
  x/1 -> IQN x IQN/1
  IQN x IQN/1 -> Kx/1

== system Final_V620140905h5b_fuben1/Function-Call Subsystem1/ION multiply5 ==
  x : Inport
  Constant2 : Constant  Value=x  OutDataTypeStr=Inherit: Inherit via back propagation
  IQN x IQN : tiiqmathlib/IQN x IQN  multiplyOption=Multiply
  Kx : Outport
  wires:
  Constant2/1 -> IQN x IQN/2
  x/1 -> IQN x IQN/1
  IQN x IQN/1 -> Kx/1

== system Final_V620140905h5b_fuben1/Function-Call Subsystem1/ION multiply6 ==
  x : Inport
  Constant2 : Constant  Value=x  OutDataTypeStr=fixdt(1,32,16)
  IQN x IQN : tiiqmathlib/IQN x IQN  multiplyOption=Multiply
  Kx : Outport
  wires:
  Constant2/1 -> IQN x IQN/2
  x/1 -> IQN x IQN/1
  IQN x IQN/1 -> Kx/1

== system Final_V620140905h5b_fuben1/Function-Call Subsystem1/ION multiply7 ==
  x : Inport
  Constant2 : Constant  Value=x  OutDataTypeStr=fixdt(1,32,16)
  IQN x IQN : tiiqmathlib/IQN x IQN  multiplyOption=Multiply
  Kx : Outport
  wires:
  Constant2/1 -> IQN x IQN/2
  x/1 -> IQN x IQN/1
  IQN x IQN/1 -> Kx/1

== system Final_V620140905h5b_fuben1/Function-Call Subsystem1/ION multiply8 ==
  x : Inport
  Constant2 : Constant  Value=x  OutDataTypeStr=fixdt(1,32,16)
  IQN x IQN : tiiqmathlib/IQN x IQN  multiplyOption=Multiply
  Kx : Outport
  wires:
  IQN x IQN/1 -> Kx/1
  x/1 -> IQN x IQN/1
  Constant2/1 -> IQN x IQN/2

== system Final_V620140905h5b_fuben1/Function-Call Subsystem1/ION multiply9 ==
  x : Inport
  Constant2 : Constant  Value=x  OutDataTypeStr=fixdt(1,32,16)
  IQN x IQN : tiiqmathlib/IQN x IQN  multiplyOption=Multiply
  Kx : Outport
  wires:
  Constant2/1 -> IQN x IQN/2
  x/1 -> IQN x IQN/1
  IQN x IQN/1 -> Kx/1

== system Final_V620140905h5b_fuben1/Function-Call Subsystem1/Integration 0 to maximal ==
  x : Inport
  3 : Constant  Value=a  OutDataTypeStr=fixdt(1,32,16)
  Relational Operator1 : RelationalOperator  Operator=<=
  Sum1 : Sum  Inputs=+-
  Sum2 : Sum
  Switch2 : Switch  Criteria=u2 > Threshold  SaturateOnIntegerOverflow=on  InputSameDT=on
  Unit Delay1 : UnitDelay  SampleTime=-1
  y : Outport
  Zero Trig : Outport  Port=2
  wires:
  Unit Delay1/1 -> Sum2/1
  Sum2/1 -> Switch2/1, Relational Operator1/1, Sum1/1
  3/1 -> Relational Operator1/2, Sum1/2
  Relational Operator1/1 -> Switch2/2, Zero Trig/1
  Switch2/1 -> Unit Delay1/1, y/1
  Sum1/1 -> Switch2/3
  x/1 -> Sum2/2

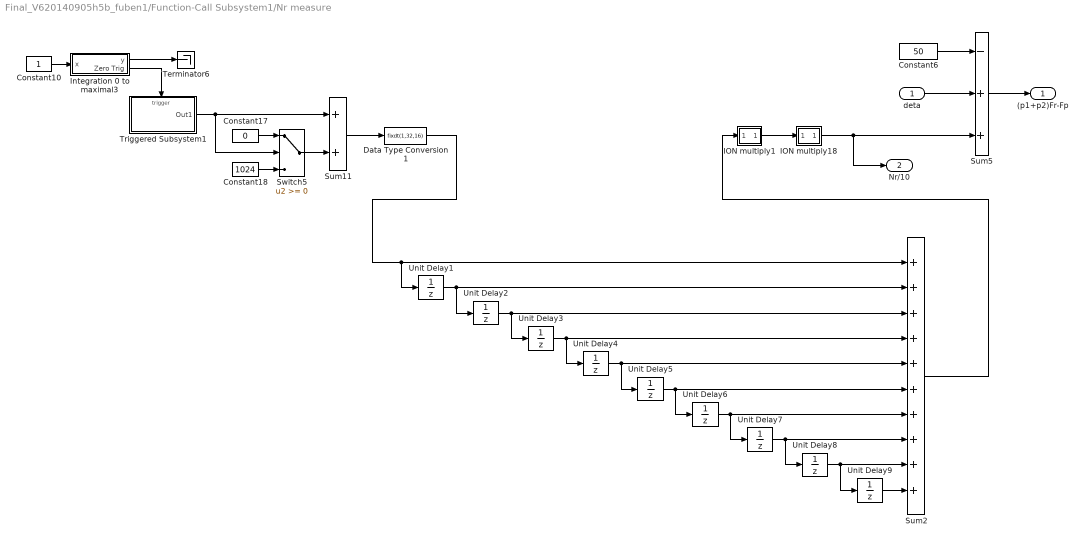
== system Final_V620140905h5b_fuben1/Function-Call Subsystem1/Nr measure ==
  deta : Inport
  Constant10 : Constant  OutDataTypeStr=fixdt(1,32,16)
  Constant17 : Constant  Value=0  OutDataTypeStr=int16
  Constant18 : Constant  Value=1024  OutDataTypeStr=int16
  Constant6 : Constant  Value=50  OutDataTypeStr=Inherit: Inherit via back propagation
  Data Type Conversion1 : DataTypeConversion  OutDataTypeStr=fixdt(1,32,16)
  ION multiply1 : Subsystem  mask{x=1/10}
      mask prompts: x "gain"
  ION multiply18 : Subsystem  mask{x=6/300/1024*5000}
      mask prompts: x "gain"
  Integration 0 to maximal3 : Subsystem  mask{a=300}
      mask prompts: a "the maximal y"
  Sum11 : Sum  AccumDataTypeStr=int16
  Sum2 : Sum  Inputs=++++++++++
  Sum5 : Sum  Inputs=-++
  Switch5 : Switch  OutDataTypeStr=int16  SaturateOnIntegerOverflow=on  InputSameDT=on
  Terminator6 : Terminator
  Triggered Subsystem1 : Subsystem  TreatAsAtomicUnit=on
  Unit Delay{1..9} (9 alike) : UnitDelay  SampleTime=-1
  (p1+p2)Fr-Fp : Outport
  Nr/10 : Outport  Port=2
  wires:
  Triggered Subsystem1/1(Out1) -> Sum11/1, Switch5/2
  Constant17/1 -> Switch5/1
  Constant18/1 -> Switch5/3
  Switch5/1 -> Sum11/2
  Constant10/1 -> Integration 0 to maximal3/1(x)
  Integration 0 to maximal3/2(Zero Trig) -> Triggered Subsystem1/Trigger
  Constant6/1 -> Sum5/1
  ION multiply18/1(Kx) -> Sum5/3, Nr/10/1
  Integration 0 to maximal3/1(y) -> Terminator6/1
  Sum5/1 -> (p1+p2)Fr-Fp/1
  deta/1 -> Sum5/2
  Sum11/1 -> Data Type Conversion1/1
  Data Type Conversion1/1 -> Unit Delay1/1, Sum2/1
  Unit Delay1/1 -> Unit Delay2/1, Sum2/2
  Unit Delay3/1 -> Unit Delay4/1, Sum2/4
  Unit Delay4/1 -> Unit Delay5/1, Sum2/5
  Unit Delay2/1 -> Unit Delay3/1, Sum2/3
  Unit Delay5/1 -> Sum2/6, Unit Delay6/1
  Sum2/1 -> ION multiply1/1(x)
  ION multiply1/1(Kx) -> ION multiply18/1(x)
  Unit Delay6/1 -> Sum2/7, Unit Delay7/1
  Unit Delay7/1 -> Sum2/8, Unit Delay8/1
  Unit Delay8/1 -> Sum2/9, Unit Delay9/1
  Unit Delay9/1 -> Sum2/10

== system Final_V620140905h5b_fuben1/Function-Call Subsystem1/Nr protect ==
  Trig : Inport
  Nr : Inport  Port=2
  Constant11 : Constant  Value=340  OutDataTypeStr=fixdt(1,32,16)
  Constant2 : Constant  Value=715  OutDataTypeStr=fixdt(1,32,16)
  Constant7 : Constant  Value=50  OutDataTypeStr=fixdt(1,32,16)
  ION multiply2 : Subsystem  mask{x=0.001}
      mask prompts: x "gain"
  ION multiply3 : Subsystem  mask{x=750/1511}
      mask prompts: x "gain"
  Logical Operator13 : Logic  Operator=OR  AllPortsSameDT=off  OutDataTypeStr=boolean
  Relational Operator1 : RelationalOperator
  Relational Operator2 : RelationalOperator  Operator=<=
  Relational Operator3 : RelationalOperator
  Triggered Subsystem1 : Subsystem  TreatAsAtomicUnit=on
  sample per n times : Subsystem  mask{n=200*10}
      mask prompts: n "Counter time n"
  Over_Nr : Outport
  wires:
  Constant11/1 -> Relational Operator1/1
  sample per n times/1(sum) -> Relational Operator1/2, Relational Operator3/1
  Triggered Subsystem1/1(Count1) -> Relational Operator2/2
  Constant7/1 -> Relational Operator2/1
  ION multiply2/1(Kx) -> ION multiply3/1(x)
  Constant2/1 -> Relational Operator3/2
  Relational Operator1/1 -> Logical Operator13/1
  Relational Operator3/1 -> Logical Operator13/2
  Logical Operator13/1 -> Triggered Subsystem1/1(Reset1)
  ION multiply3/1(Kx) -> sample per n times/1(x)
  Trig/1 -> Triggered Subsystem1/Trigger
  Nr/1 -> ION multiply2/1(x)
  Relational Operator2/1 -> Over_Nr/1

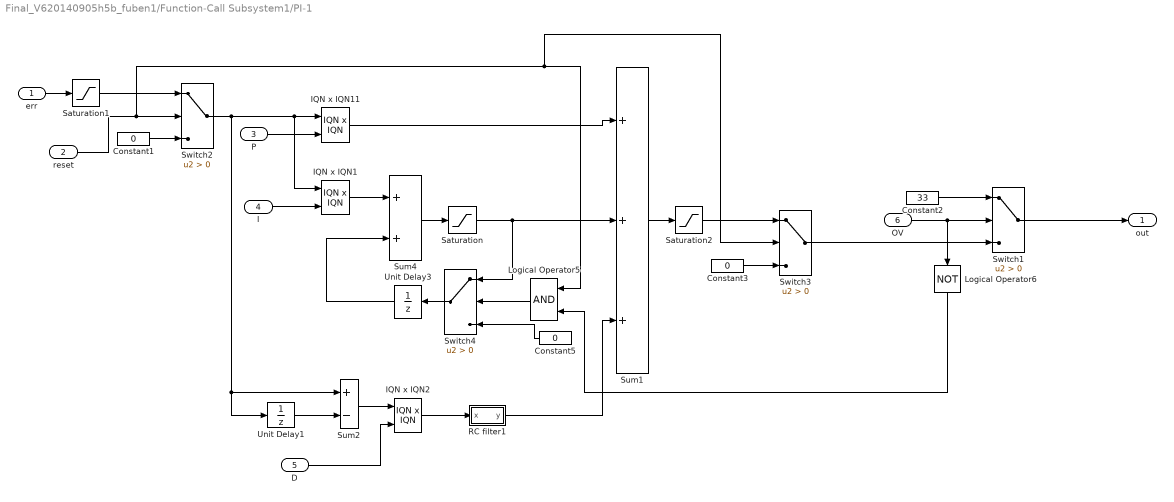
== system Final_V620140905h5b_fuben1/Function-Call Subsystem1/PI-1 ==
  err : Inport
  reset : Inport  Port=2
  P : Inport  Port=3
  I : Inport  Port=4
  D : Inport  Port=5
  OV : Inport  Port=6
  Constant1 : Constant  Value=0  OutDataTypeStr=Inherit: Inherit via back propagation
  Constant2 : Constant  Value=33  OutDataTypeStr=Inherit: Inherit via back propagation
  Constant3 : Constant  Value=0  OutDataTypeStr=Inherit: Inherit via back propagation
  Constant5 : Constant  Value=0  OutDataTypeStr=Inherit: Inherit via back propagation
  IQN x IQN1 : tiiqmathlib/IQN x IQN  multiplyOption=Multiply
  IQN x IQN11 : tiiqmathlib/IQN x IQN  multiplyOption=Multiply
  IQN x IQN2 : tiiqmathlib/IQN x IQN  multiplyOption=Multiply
  Logical Operator5 : Logic  AllPortsSameDT=off  OutDataTypeStr=boolean
  Logical Operator6 : Logic  Operator=NOT  AllPortsSameDT=off  OutDataTypeStr=boolean
  RC filter1 : Subsystem  mask{a=0.4}
      mask prompts: a "Time Constant"
  Saturation : Saturate  UpperLimit=max  LowerLimit=min  LinearizeAsGain=off  ZeroCross=off  OutDataTypeStr=fixdt(1,32,16)
  Saturation1 : Saturate  UpperLimit=ermax  LowerLimit=ermin  LinearizeAsGain=off  ZeroCross=off  OutDataTypeStr=fixdt(1,32,16)
  Saturation2 : Saturate  UpperLimit=max  LowerLimit=min  LinearizeAsGain=off  ZeroCross=off  OutDataTypeStr=fixdt(1,32,16)
  Sum1 : Sum  Inputs=+++
  Sum2 : Sum  Inputs=+-
  Sum4 : Sum
  Switch{1..4} (4 alike) : Switch  Criteria=u2 > Threshold  SaturateOnIntegerOverflow=on  InputSameDT=on
  Unit Delay1 : UnitDelay  SampleTime=-1
  Unit Delay3 : UnitDelay  SampleTime=-1
  out : Outport
  wires:
  Logical Operator6/1 -> Logical Operator5/2
  Logical Operator5/1 -> Switch4/2
  RC filter1/1(y) -> Sum1/3
  Constant3/1 -> Switch3/3
  Switch3/1 -> Switch1/3
  Saturation2/1 -> Switch3/1
  Switch1/1 -> out/1
  OV/1 -> Logical Operator6/1, Switch1/2
  Constant2/1 -> Switch1/1
  Sum1/1 -> Saturation2/1
  IQN x IQN2/1 -> RC filter1/1(x)
  Unit Delay1/1 -> Sum2/2
  D/1 -> IQN x IQN2/2
  Sum2/1 -> IQN x IQN2/1
  Switch4/1 -> Unit Delay3/1
  Unit Delay3/1 -> Sum4/2
  Saturation/1 -> Switch4/1, Sum1/2
  Sum4/1 -> Saturation/1
  IQN x IQN1/1 -> Sum4/1
  I/1 -> IQN x IQN1/2
  IQN x IQN11/1 -> Sum1/1
  Saturation1/1 -> Switch2/1
  err/1 -> Saturation1/1
  Constant1/1 -> Switch2/3
  reset/1 -> Logical Operator5/1, Switch3/2, Switch2/2
  Switch2/1 -> Unit Delay1/1, Sum2/1, IQN x IQN1/1, IQN x IQN11/1
  P/1 -> IQN x IQN11/2
  Constant5/1 -> Switch4/3

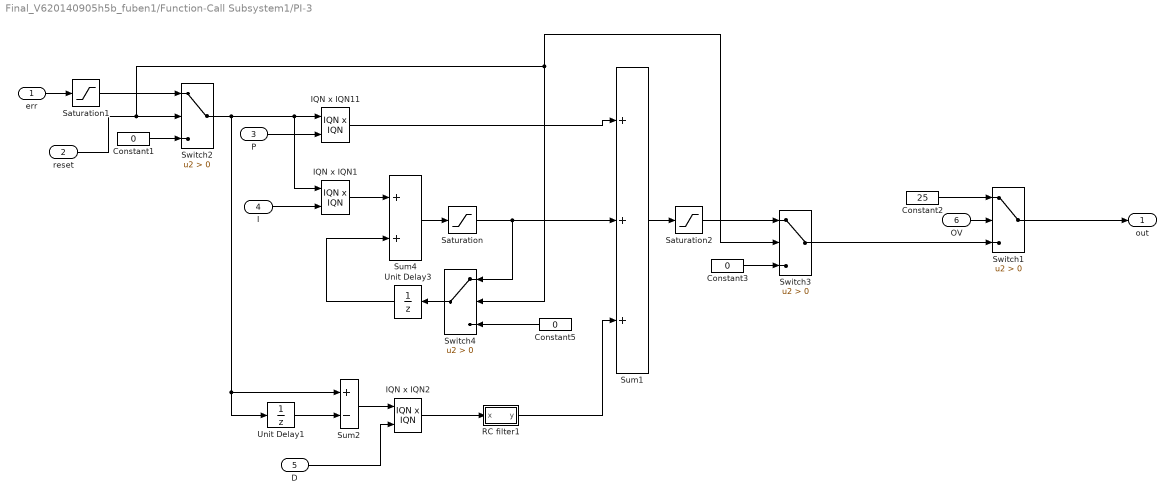
== system Final_V620140905h5b_fuben1/Function-Call Subsystem1/PI-3 ==
  err : Inport
  reset : Inport  Port=2
  P : Inport  Port=3
  I : Inport  Port=4
  D : Inport  Port=5
  OV : Inport  Port=6
  Constant1 : Constant  Value=0  OutDataTypeStr=Inherit: Inherit via back propagation
  Constant2 : Constant  Value=25  OutDataTypeStr=Inherit: Inherit via back propagation
  Constant3 : Constant  Value=0  OutDataTypeStr=Inherit: Inherit via back propagation
  Constant5 : Constant  Value=0  OutDataTypeStr=Inherit: Inherit via back propagation
  IQN x IQN1 : tiiqmathlib/IQN x IQN  multiplyOption=Multiply
  IQN x IQN11 : tiiqmathlib/IQN x IQN  multiplyOption=Multiply
  IQN x IQN2 : tiiqmathlib/IQN x IQN  multiplyOption=Multiply
  RC filter1 : Subsystem  mask{a=0.4}
      mask prompts: a "Time Constant"
  Saturation : Saturate  UpperLimit=max  LowerLimit=min  LinearizeAsGain=off  ZeroCross=off  OutDataTypeStr=fixdt(1,32,16)
  Saturation1 : Saturate  UpperLimit=ermax  LowerLimit=ermin  LinearizeAsGain=off  ZeroCross=off  OutDataTypeStr=fixdt(1,32,16)
  Saturation2 : Saturate  UpperLimit=max  LowerLimit=min  LinearizeAsGain=off  ZeroCross=off  OutDataTypeStr=fixdt(1,32,16)
  Sum1 : Sum  Inputs=+++
  Sum2 : Sum  Inputs=+-
  Sum4 : Sum
  Switch{1..4} (4 alike) : Switch  Criteria=u2 > Threshold  SaturateOnIntegerOverflow=on  InputSameDT=on
  Unit Delay1 : UnitDelay  SampleTime=-1
  Unit Delay3 : UnitDelay  SampleTime=-1
  out : Outport
  wires:
  RC filter1/1(y) -> Sum1/3
  Constant5/1 -> Switch4/3
  P/1 -> IQN x IQN11/2
  Switch2/1 -> IQN x IQN11/1, IQN x IQN1/1, Sum2/1, Unit Delay1/1
  reset/1 -> Switch2/2, Switch4/2, Switch3/2
  Constant1/1 -> Switch2/3
  err/1 -> Saturation1/1
  Saturation1/1 -> Switch2/1
  IQN x IQN11/1 -> Sum1/1
  I/1 -> IQN x IQN1/2
  IQN x IQN1/1 -> Sum4/1
  Sum4/1 -> Saturation/1
  Saturation/1 -> Sum1/2, Switch4/1
  Unit Delay3/1 -> Sum4/2
  Switch4/1 -> Unit Delay3/1
  Sum2/1 -> IQN x IQN2/1
  D/1 -> IQN x IQN2/2
  Unit Delay1/1 -> Sum2/2
  IQN x IQN2/1 -> RC filter1/1(x)
  Sum1/1 -> Saturation2/1
  Constant2/1 -> Switch1/1
  OV/1 -> Switch1/2
  Switch1/1 -> out/1
  Saturation2/1 -> Switch3/1
  Switch3/1 -> Switch1/3
  Constant3/1 -> Switch3/3

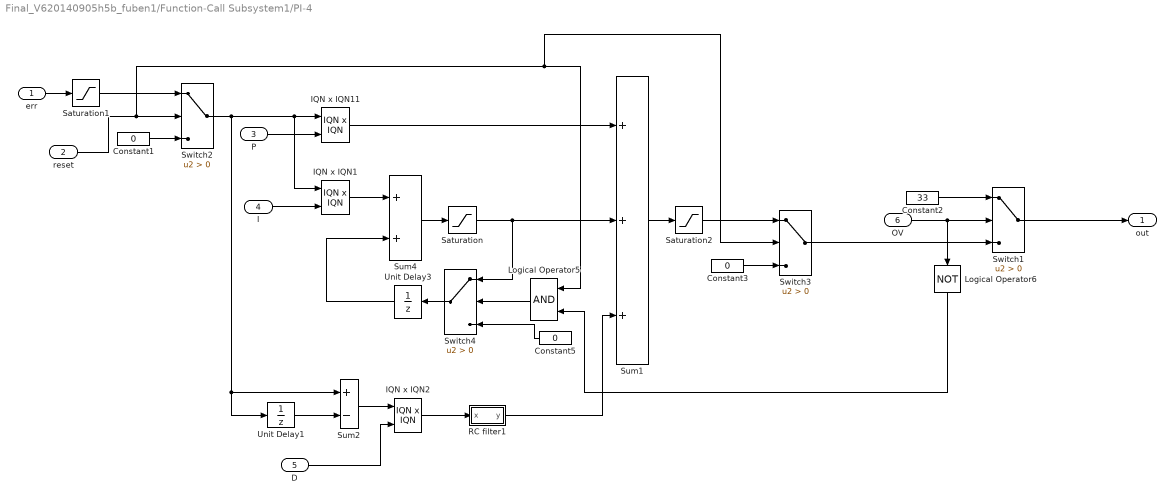
== system Final_V620140905h5b_fuben1/Function-Call Subsystem1/PI-4 ==
  err : Inport
  reset : Inport  Port=2
  P : Inport  Port=3
  I : Inport  Port=4
  D : Inport  Port=5
  OV : Inport  Port=6
  Constant1 : Constant  Value=0  OutDataTypeStr=Inherit: Inherit via back propagation
  Constant2 : Constant  Value=33  OutDataTypeStr=Inherit: Inherit via back propagation
  Constant3 : Constant  Value=0  OutDataTypeStr=Inherit: Inherit via back propagation
  Constant5 : Constant  Value=0  OutDataTypeStr=Inherit: Inherit via back propagation
  IQN x IQN1 : tiiqmathlib/IQN x IQN  multiplyOption=Multiply
  IQN x IQN11 : tiiqmathlib/IQN x IQN  multiplyOption=Multiply
  IQN x IQN2 : tiiqmathlib/IQN x IQN  multiplyOption=Multiply
  Logical Operator5 : Logic  AllPortsSameDT=off  OutDataTypeStr=boolean
  Logical Operator6 : Logic  Operator=NOT  AllPortsSameDT=off  OutDataTypeStr=boolean
  RC filter1 : Subsystem  mask{a=0.4}
      mask prompts: a "Time Constant"
  Saturation : Saturate  UpperLimit=max  LowerLimit=min  LinearizeAsGain=off  ZeroCross=off  OutDataTypeStr=fixdt(1,32,16)
  Saturation1 : Saturate  UpperLimit=ermax  LowerLimit=ermin  LinearizeAsGain=off  ZeroCross=off  OutDataTypeStr=fixdt(1,32,16)
  Saturation2 : Saturate  UpperLimit=max  LowerLimit=min  LinearizeAsGain=off  ZeroCross=off  OutDataTypeStr=fixdt(1,32,16)
  Sum1 : Sum  Inputs=+++
  Sum2 : Sum  Inputs=+-
  Sum4 : Sum
  Switch{1..4} (4 alike) : Switch  Criteria=u2 > Threshold  SaturateOnIntegerOverflow=on  InputSameDT=on
  Unit Delay1 : UnitDelay  SampleTime=-1
  Unit Delay3 : UnitDelay  SampleTime=-1
  out : Outport
  wires:
  Constant5/1 -> Switch4/3
  P/1 -> IQN x IQN11/2
  Switch2/1 -> IQN x IQN11/1, IQN x IQN1/1, Sum2/1, Unit Delay1/1
  reset/1 -> Switch2/2, Switch3/2, Logical Operator5/1
  Constant1/1 -> Switch2/3
  err/1 -> Saturation1/1
  Saturation1/1 -> Switch2/1
  IQN x IQN11/1 -> Sum1/1
  I/1 -> IQN x IQN1/2
  IQN x IQN1/1 -> Sum4/1
  Sum4/1 -> Saturation/1
  Saturation/1 -> Sum1/2, Switch4/1
  Unit Delay3/1 -> Sum4/2
  Switch4/1 -> Unit Delay3/1
  Sum2/1 -> IQN x IQN2/1
  D/1 -> IQN x IQN2/2
  Unit Delay1/1 -> Sum2/2
  IQN x IQN2/1 -> RC filter1/1(x)
  Sum1/1 -> Saturation2/1
  Constant2/1 -> Switch1/1
  OV/1 -> Switch1/2, Logical Operator6/1
  Switch1/1 -> out/1
  Saturation2/1 -> Switch3/1
  Switch3/1 -> Switch1/3
  Constant3/1 -> Switch3/3
  RC filter1/1(y) -> Sum1/3
  Logical Operator5/1 -> Switch4/2
  Logical Operator6/1 -> Logical Operator5/2

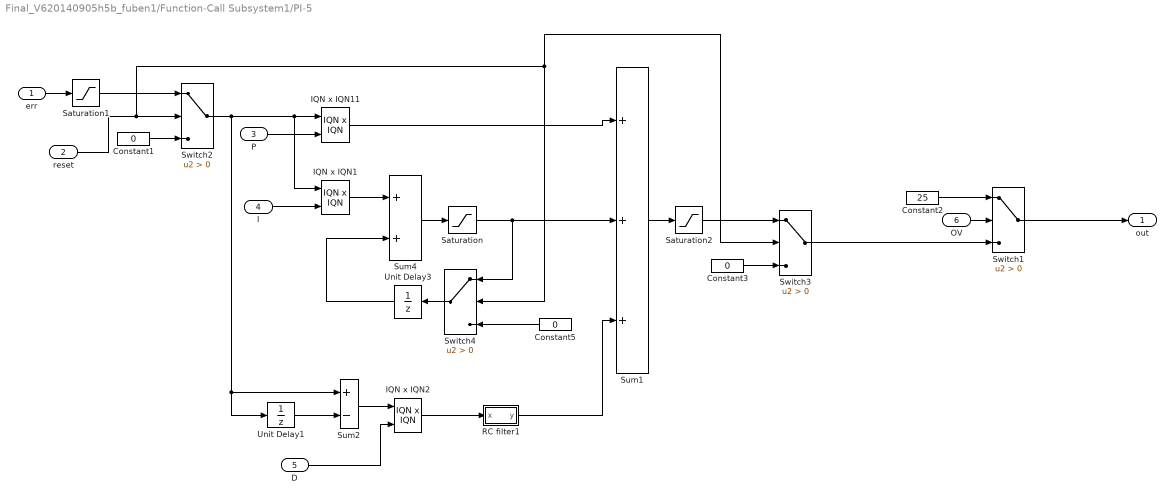
== system Final_V620140905h5b_fuben1/Function-Call Subsystem1/PI-5 ==
  err : Inport
  reset : Inport  Port=2
  P : Inport  Port=3
  I : Inport  Port=4
  D : Inport  Port=5
  OV : Inport  Port=6
  Constant1 : Constant  Value=0  OutDataTypeStr=Inherit: Inherit via back propagation
  Constant2 : Constant  Value=25  OutDataTypeStr=Inherit: Inherit via back propagation
  Constant3 : Constant  Value=0  OutDataTypeStr=Inherit: Inherit via back propagation
  Constant5 : Constant  Value=0  OutDataTypeStr=Inherit: Inherit via back propagation
  IQN x IQN1 : tiiqmathlib/IQN x IQN  multiplyOption=Multiply
  IQN x IQN11 : tiiqmathlib/IQN x IQN  multiplyOption=Multiply
  IQN x IQN2 : tiiqmathlib/IQN x IQN  multiplyOption=Multiply
  RC filter1 : Subsystem  mask{a=0.4}
      mask prompts: a "Time Constant"
  Saturation : Saturate  UpperLimit=max  LowerLimit=min  LinearizeAsGain=off  ZeroCross=off  OutDataTypeStr=fixdt(1,32,16)
  Saturation1 : Saturate  UpperLimit=ermax  LowerLimit=ermin  LinearizeAsGain=off  ZeroCross=off  OutDataTypeStr=fixdt(1,32,16)
  Saturation2 : Saturate  UpperLimit=max  LowerLimit=min  LinearizeAsGain=off  ZeroCross=off  OutDataTypeStr=fixdt(1,32,16)
  Sum1 : Sum  Inputs=+++
  Sum2 : Sum  Inputs=+-
  Sum4 : Sum
  Switch{1..4} (4 alike) : Switch  Criteria=u2 > Threshold  SaturateOnIntegerOverflow=on  InputSameDT=on
  Unit Delay1 : UnitDelay  SampleTime=-1
  Unit Delay3 : UnitDelay  SampleTime=-1
  out : Outport
  wires:
  Constant3/1 -> Switch3/3
  Switch3/1 -> Switch1/3
  Saturation2/1 -> Switch3/1
  Switch1/1 -> out/1
  OV/1 -> Switch1/2
  Constant2/1 -> Switch1/1
  Sum1/1 -> Saturation2/1
  IQN x IQN2/1 -> RC filter1/1(x)
  Unit Delay1/1 -> Sum2/2
  D/1 -> IQN x IQN2/2
  Sum2/1 -> IQN x IQN2/1
  Switch4/1 -> Unit Delay3/1
  Unit Delay3/1 -> Sum4/2
  Saturation/1 -> Switch4/1, Sum1/2
  Sum4/1 -> Saturation/1
  IQN x IQN1/1 -> Sum4/1
  I/1 -> IQN x IQN1/2
  IQN x IQN11/1 -> Sum1/1
  Saturation1/1 -> Switch2/1
  err/1 -> Saturation1/1
  Constant1/1 -> Switch2/3
  reset/1 -> Switch3/2, Switch4/2, Switch2/2
  Switch2/1 -> Unit Delay1/1, Sum2/1, IQN x IQN1/1, IQN x IQN11/1
  P/1 -> IQN x IQN11/2
  Constant5/1 -> Switch4/3
  RC filter1/1(y) -> Sum1/3

== system Final_V620140905h5b_fuben1/Function-Call Subsystem1/RC filter10 ==
  x : Inport
  Constant2 : Constant  Value=a  OutDataTypeStr=fixdt(1,32,16)
  Constant3 : Constant  Value=1-a  OutDataTypeStr=fixdt(1,32,16)
  IQN x IQN : tiiqmathlib/IQN x IQN  multiplyOption=Multiply
  IQN x IQN1 : tiiqmathlib/IQN x IQN  multiplyOption=Multiply
  Sum2 : Sum
  Unit Delay2 : UnitDelay  SampleTime=-1
  y : Outport
  wires:
  Unit Delay2/1 -> IQN x IQN1/2
  Sum2/1 -> Unit Delay2/1, y/1
  IQN x IQN1/1 -> Sum2/2
  IQN x IQN/1 -> Sum2/1
  Constant3/1 -> IQN x IQN1/1
  Constant2/1 -> IQN x IQN/2
  x/1 -> IQN x IQN/1

== system Final_V620140905h5b_fuben1/Function-Call Subsystem1/RC filter11 ==
  x : Inport
  Constant2 : Constant  Value=a  OutDataTypeStr=fixdt(1,32,16)
  Constant3 : Constant  Value=1-a  OutDataTypeStr=fixdt(1,32,16)
  IQN x IQN : tiiqmathlib/IQN x IQN  multiplyOption=Multiply
  IQN x IQN1 : tiiqmathlib/IQN x IQN  multiplyOption=Multiply
  Sum2 : Sum
  Unit Delay2 : UnitDelay  SampleTime=-1
  y : Outport
  wires:
  x/1 -> IQN x IQN/1
  Constant2/1 -> IQN x IQN/2
  Constant3/1 -> IQN x IQN1/1
  IQN x IQN/1 -> Sum2/1
  IQN x IQN1/1 -> Sum2/2
  Sum2/1 -> y/1, Unit Delay2/1
  Unit Delay2/1 -> IQN x IQN1/2

== system Final_V620140905h5b_fuben1/Function-Call Subsystem1/RC filter15 ==
  x : Inport
  Constant2 : Constant  Value=a  OutDataTypeStr=fixdt(1,32,16)
  Constant3 : Constant  Value=1-a  OutDataTypeStr=fixdt(1,32,16)
  IQN x IQN : tiiqmathlib/IQN x IQN  multiplyOption=Multiply
  IQN x IQN1 : tiiqmathlib/IQN x IQN  multiplyOption=Multiply
  Sum2 : Sum
  Unit Delay2 : UnitDelay  SampleTime=-1
  y : Outport
  wires:
  Unit Delay2/1 -> IQN x IQN1/2
  Sum2/1 -> Unit Delay2/1, y/1
  IQN x IQN1/1 -> Sum2/2
  IQN x IQN/1 -> Sum2/1
  Constant3/1 -> IQN x IQN1/1
  Constant2/1 -> IQN x IQN/2
  x/1 -> IQN x IQN/1
